simulink model "tank_reglering_PID"  (R2017b)
settings: Solver=VariableStepAuto  StartTime=0.0  StopTime=inf  RelTol=1e-3
values from neighbouring files (symbols this model uses):
  k = K8*Tf/Td    [PIDdesign.m]
  Td = (sqrt(my*(my-cos(PhiR)))+my*sin(PhiR))/(2*wc*(my*cos(PhiR)-1))    [PIDdesign.m]
  Tf = Td*cos(PhiR)/(my+wc*Td*sin(PhiR))    [PIDdesign.m]
  Ti = 4*Td    [PIDdesign.m]
undefined symbols (not defined in the file or in its folder): H, Y
libraries: Tank_bib x1
settings Model: Creator=Oliver  LastModifiedBy=Oliver

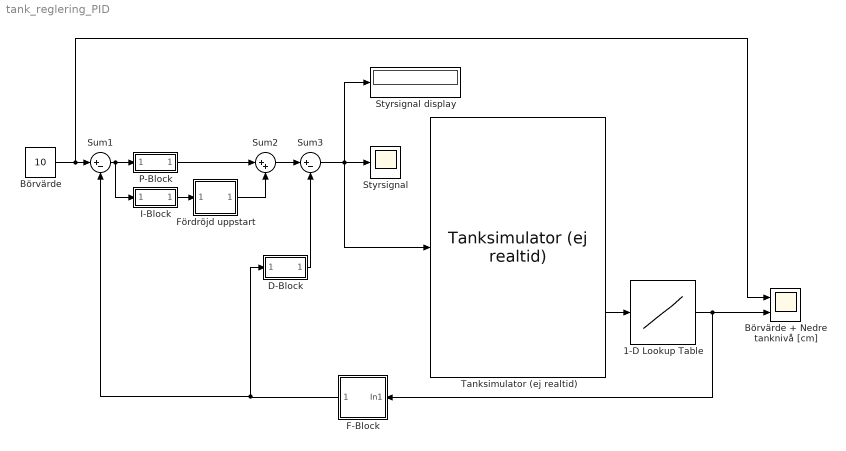
== system tank_reglering_PID ==
  1-D Lookup Table : Lookup_n-D  NumberOfTableDimensions=1  BreakpointsForDimension1=Y  Table=H  InternalRulePriority=Speed  RndMeth=Simplest  InputSameDT=on
  Börvärde : Constant  Value=10
  Börvärde + Nedre tanknivå [cm] : Scope  NumInputPorts=2
  D-Block : Subsystem
  F-Block : Subsystem
  Fördröjd uppstart : Subsystem
  I-Block : Subsystem
  P-Block : Subsystem
  Styrsignal : Scope
  Styrsignal display : Display
  Sum1 : Sum  Inputs=|+-
  Sum2 : Sum  Inputs=|++
  Sum3 : Sum  Inputs=|+-
  Tanksimulator (ej realtid) : Tank_bib/Tanksimulator (ej realtid)  valve_opening=0  plug=off
  wires:
  Börvärde/1 -> Börvärde + Nedre tanknivå [cm]/1, Sum1/1
  Sum3/1 -> Styrsignal display/1, Tanksimulator (ej realtid)/1, Styrsignal/1
  P-Block/1(Out1) -> Sum2/1
  Sum2/1 -> Sum3/1
  Sum1/1 -> I-Block/1(In1), P-Block/1(In1)
  D-Block/1(Out1) -> Sum3/2
  Tanksimulator (ej realtid)/2 -> 1-D Lookup Table/1
  1-D Lookup Table/1 -> Börvärde + Nedre tanknivå [cm]/2, F-Block/1(In1)
  F-Block/1(Out1) -> D-Block/1(In1), Sum1/2
  I-Block/1(Out1) -> Fördröjd uppstart/1(In1)
  Fördröjd uppstart/1(Out1) -> Sum2/2

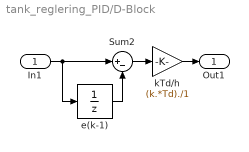
== system tank_reglering_PID/D-Block ==
  In1 : Inport
  Sum2 : Sum  Inputs=|+-
  e(k-1) : UnitDelay  SampleTime=-1
  kTd/h : Gain  Gain=(k.*Td)./1
  Out1 : Outport
  wires:
  Sum2/1 -> kTd/h/1
  kTd/h/1 -> Out1/1
  e(k-1)/1 -> Sum2/2
  In1/1 -> e(k-1)/1, Sum2/1

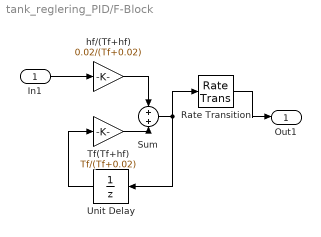
== system tank_reglering_PID/F-Block ==
  In1 : Inport
  Rate Transition : RateTransition  OutPortSampleTime=1
  Sum : Sum  Inputs=+|+
  Tf(Tf+hf) : Gain  Gain=Tf/(Tf+0.02)
  Unit Delay : UnitDelay  SampleTime=-1
  hf/(Tf+hf) : Gain  Gain=0.02/(Tf+0.02)
  Out1 : Outport
  wires:
  Unit Delay/1 -> Tf(Tf+hf)/1
  In1/1 -> hf/(Tf+hf)/1
  hf/(Tf+hf)/1 -> Sum/1
  Tf(Tf+hf)/1 -> Sum/2
  Sum/1 -> Unit Delay/1, Rate Transition/1
  Rate Transition/1 -> Out1/1

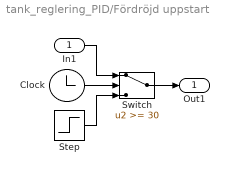
== system tank_reglering_PID/Fördröjd uppstart ==
  In1 : Inport
  Clock : Clock
  Step : Step  After=k  SampleTime=0
  Switch : Switch  Threshold=30
  Out1 : Outport
  wires:
  Clock/1 -> Switch/2
  Switch/1 -> Out1/1
  In1/1 -> Switch/1
  Step/1 -> Switch/3

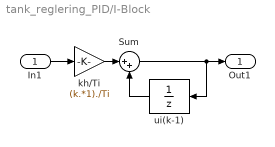
== system tank_reglering_PID/I-Block ==
  In1 : Inport
  Sum : Sum  Inputs=|++
  kh/Ti : Gain  Gain=(k.*1)./Ti
  ui(k-1) : UnitDelay  SampleTime=-1
  Out1 : Outport
  wires:
  In1/1 -> kh/Ti/1
  kh/Ti/1 -> Sum/1
  ui(k-1)/1 -> Sum/2
  Sum/1 -> ui(k-1)/1, Out1/1

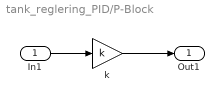
== system tank_reglering_PID/P-Block ==
  In1 : Inport
  k : Gain  Gain=k
  Out1 : Outport
  wires:
  In1/1 -> k/1
  k/1 -> Out1/1
